simulink model "MYmotoSys1b_centrifugal"  (R2021a)
settings: Solver=ode45  StartTime=0.0  StopTime=20  RelTol=1e-3  EnableMultiTasking=on
PreLoadFcn:
  | moto_cad_data
  | 
  | theta0 = 1;
  | thetadot0 = 0;
undefined symbols (not defined in the file): magnitude, smiData_bike_body, smiData_front_wheel, smiData_reaction_wheel, smiData_rear_wheel, smiData_steer_column, X, Y, Z
libraries: sm_lib x18, nesl_utility x7
settings Model: EnablePacing=on  Creator=smiller  LastModifiedBy=danie
settings SolverCC: AlgebraicLoopSolver=TrustRegion
settings DataIOCC: LimitDataPoints=on  SaveFormat=Array  ReturnWorkspaceOutputs=off
settings OptimizationCC: ExpressionDepthLimit=2147483647  LifeSpan=inf
settings DebuggingCC: UnderspecifiedInitializationDetection=Classic  MergeDetectMultiDrivingBlocksExec=none  ParameterPrecisionLossMsg=none  StateNameClashWarn=warning  SFUnexpectedBacktrackingDiag=warning  SFNoUnconditionalDefaultTransitionDiag=warning  SFExecutionAtInitializationDiag=none  SFMachineParentedDataDiag=warning  ArithmeticOperatorsInVariantConditions=warning
settings HardwareCC: ProdBitPerPointer=32  ProdBitPerSizeT=32  ProdBitPerPtrDiffT=32  ProdLargestAtomicFloat=None  ProdIntDivRoundTo=Undefined  ProdEndianess=Unspecified  ProdWordSize=32  ProdHWDeviceType=32-bit Generic
settings ModelReferenceCC: PropagateSignalLabelsOutOfModel=off
settings SFSimCC: SimUseLocalCustomCode=off  CustomCodeUndefinedFunction=UseInterfaceOnly
settings RTWCC: RTWUseLocalCustomCode=off
settings CodeAppCC: StateflowObjectComments=on
settings GRTTargetCC: TargetLangStandard=C89/C90 (ANSI)
settings ConfigComp: CovMetricSettings=dw  CovSaveCumulativeToWorkspaceVar=on  CovSaveSingleToWorkspaceVar=on  CovExternalEMLEnable=off  CovSFcnEnable=off
settings SimscapeCC: SimscapeNormalizeSystem=off
settings ConfigurationSet: Description=SimMechanics 2G
settings ExplorerConfigSet: InternalSimMechanicsExplorerSettings="<ExplorerConfiguration><canonicalview>default</canonicalview><AnimationSetting><BasePlaybackSpeed>1.0</BasePlaybackSpeed><PlaybackSpeedFactor>1.0</PlaybackSpeedFactor></AnimationSetting><TilePanel><TileInfo><Tiles Columns=\"1\" Count=\"1\" Rows=\"1\"><Column Weight=\"1\"/><Row Weight=\"1\"/><Tile Height=\"1\" Width=\"1\" X=\"0\" Y=\"0\"/></Tiles></TileInfo><SceneInfo><SceneViewer><BGColor><R>0.60000002384185791</R><G>0.60000002384185791</G><B>0.60000002384185791</B></BGColor><Camera><DoPerspective>off</DoPerspective><Position><X>0.918124572942673689</X><Y>-0.460889112225935038</Y><Z>0.271893212526261863</Z></Position><Center><X>0.0428283947711830537</X><Y>-0.012621623404857174</Y><Z>0.090474197689223379</Z></Center><Up><X>-0.135786056615979422</X><Y>0.132236903462622957</Y><Z>0.981873488893196922</Z></Up><ViewLimDist>1</ViewLimDist><YLim>0.105450724735856052</YLim><XLim>0.181023744129886199</XLim></Camera></SceneViewer></SceneInfo></TilePanel><MechEditorPanel><Cameras/><GfxPanelCameraMap/><VideoCreator><PlaybackSpeedRatio>1.0</PlaybackSpeedRatio><FrameRate>30</FrameRate><VideoFormat>Motion JPEG AVI</VideoFormat><FrameSize>auto</FrameSize></VideoCreator></MechEditorPanel></ExplorerConfiguration>"

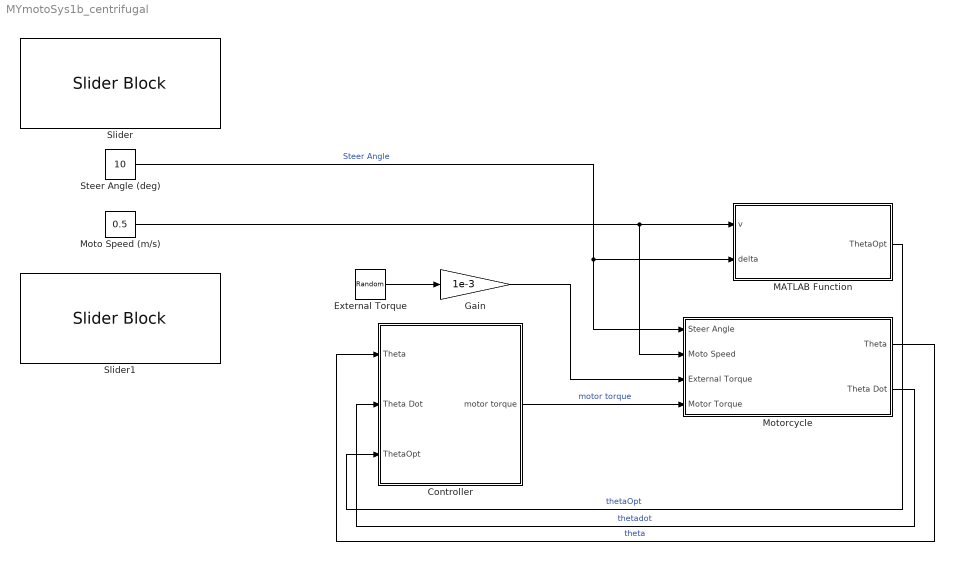
== system MYmotoSys1b_centrifugal ==
  Controller : Subsystem
  External Torque : RandomNumber  SampleTime=0.1
  Gain : Gain  Gain=1e-3
  MATLAB Function : MATLAB Function  TreatAsAtomicUnit=on
  Moto Speed (m/s) : Constant  Value=0.5  SampleTime=-1
  Motorcycle : Subsystem
  Slider : SliderBlock  ScaleMin=-30  ScaleMax=30
  Slider1 : SliderBlock  ScaleMin=-2  ScaleMax=2
  Steer Angle (deg) : Constant  Value=10  SampleTime=-1
  wires:
  Motorcycle/1(Theta) -> Controller/1(Theta)  "theta"
  Motorcycle/2(Theta Dot) -> Controller/2(Theta Dot)  "thetadot"
  External Torque/1 -> Gain/1
  Gain/1 -> Motorcycle/3(External Torque)
  Moto Speed (m/s)/1 -> MATLAB Function/1(v), Motorcycle/2(Moto Speed)
  Steer Angle (deg)/1 -> MATLAB Function/2(delta), Motorcycle/1(Steer Angle)  "Steer Angle"
  Controller/1(motor torque) -> Motorcycle/4(Motor Torque)  "motor torque"
  MATLAB Function/1(ThetaOpt) -> Controller/3(ThetaOpt)  "thetaOpt"

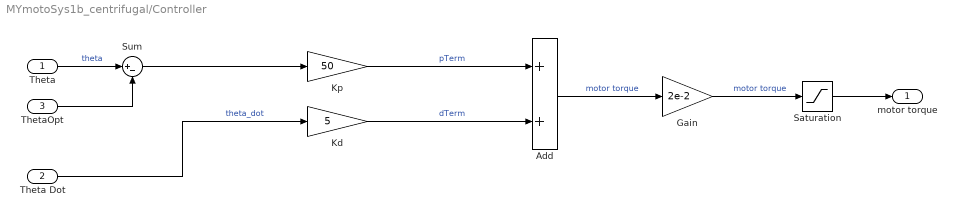
== system MYmotoSys1b_centrifugal/Controller ==
  Theta : Inport
  Theta Dot : Inport  Port=2
  ThetaOpt : Inport  Port=3
  Add : Sum  Inputs=2
  "Gain " : Gain  Gain=2e-2
  Kd : Gain  Gain=5
  Kp : Gain  Gain=50
  Saturation : Saturate  UpperLimit=0.7  LowerLimit=-0.7
  Sum : Sum  Inputs=|+-
  motor torque : Outport  VectorParamsAs1DForOutWhenUnconnected=off
  wires:
  Kd/1 -> Add/2  "dTerm"
  "Gain "/1 -> Saturation/1  "motor torque"
  Kp/1 -> Add/1  "pTerm"
  Theta/1 -> Sum/1  "theta"
  Add/1 -> "Gain "/1  "motor torque"
  Theta Dot/1 -> Kd/1  "theta_dot"
  ThetaOpt/1 -> Sum/2
  Sum/1 -> Kp/1
  Saturation/1 -> motor torque/1

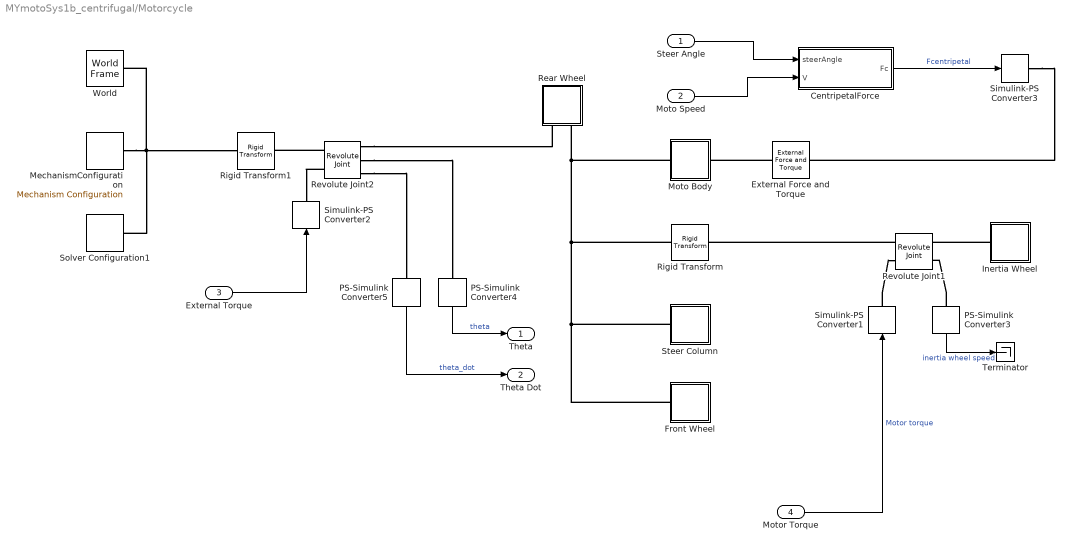
== system MYmotoSys1b_centrifugal/Motorcycle ==
  Steer Angle : Inport
  Moto Speed : Inport  Port=2
  External Torque : Inport  Port=3
  Motor Torque : Inport  Port=4
  CentripetalForce : Subsystem
  External Force and Torque : sm_lib/Forces and Torques/External Force and Torque  ForceResolutionFrame=AttachedFrame  EnableForceX=off  EnableForceY=on  EnableForceZ=off  EnableForce=off  TorqueResolutionFrame=AttachedFrame  EnableTorqueX=off  EnableTorqueY=off  EnableTorqueZ=off  EnableTorque=off
  Front Wheel : Subsystem
  Inertia Wheel : Subsystem
  MechanismConfiguration : sm_lib/Utilities/Mechanism Configuration  UniformGravity=Constant  GravityVector=[0 0 -9.80665]  GravityVectorUnits=m/s^2  GravityUnits=m/s^2  LinearizationDelta=0.001  JointModeTransitionNonlinearIterations=2
  Moto Body : Subsystem
  PS-Simulink Converter3 : nesl_utility/PS-Simulink Converter  PhysicalDomain=network_engine_domain  SubClassName=ps_output  LeftPortType=input  RightPortType=output  PseudoPeriodic=off  Frequencies=[]  Unit=rev/s  AffineConversion=off
      settings: SourceProductBaseCode=PW,SS
  PS-Simulink Converter4 : nesl_utility/PS-Simulink Converter  PhysicalDomain=network_engine_domain  SubClassName=ps_output  LeftPortType=input  RightPortType=output  PseudoPeriodic=off  Frequencies=[]  Unit=deg  AffineConversion=off
      settings: SourceProductBaseCode=PW,SS
  PS-Simulink Converter5 : nesl_utility/PS-Simulink Converter  PhysicalDomain=network_engine_domain  SubClassName=ps_output  LeftPortType=input  RightPortType=output  PseudoPeriodic=off  Frequencies=[]  Unit=deg/s  AffineConversion=off
      settings: SourceProductBaseCode=PW,SS
  Rear Wheel : Subsystem
  Revolute Joint1 : sm_lib/Joints/Revolute Joint  JointMode=Normal  SenseConstraintForce=off  SenseConstraintForceX=off  SenseConstraintForceY=off  SenseConstraintForceZ=off  SenseConstraintTorque=off  SenseConstraintTorqueX=off  SenseConstraintTorqueY=off  SenseConstraintTorqueZ=off  SenseTotalForce=off  SenseTotalForceX=off  SenseTotalForceY=off  SenseTotalForceZ=off  SenseTotalTorque=off  SenseTotalTorqueX=off  SenseTotalTorqueY=off  SenseTotalTorqueZ=off  CompositeWrenchDir=FollowerOnBase  CompositeWrenchFrame=BaseFrame  EquilibriumPosition=0  EquilibriumPositionUnits=deg  SpringStiffness=0  SpringStiffnessUnits=N*m/deg  DampingCoefficient=0  DampingCoefficientUnits=N*m/(deg/s)  TorqueActuationMode=InputTorque  MotionActuationMode=ComputedMotion  SensePosition=off  SenseVelocity=on  SenseAcceleration=off  SenseTorqueForce=off  SenseLowerLimitTorqueForce=off  SenseUpperLimitTorqueForce=off  LowerLimitSpecify=off  LowerLimitBound=-90  LowerLimitBoundUnits=deg  LowerLimitStiffness=1e4  LowerLimitStiffnessUnits=N*m/deg  LowerLimitDamping=10  LowerLimitDampingUnits=N*m/(deg/s)  LowerLimitTransitionRegionWidth=0.1  LowerLimitTransitionRegionWidthUnits=deg  UpperLimitSpecify=off  UpperLimitBound=90  UpperLimitBoundUnits=deg  UpperLimitStiffness=1e4  UpperLimitStiffnessUnits=N*m/deg  UpperLimitDamping=10  UpperLimitDampingUnits=N*m/(deg/s)  UpperLimitTransitionRegionWidth=0.1  UpperLimitTransitionRegionWidthUnits=deg  PositionTargetSpecify=off  PositionTargetPriority=High  PositionTargetValue=0  PositionTargetValueUnits=deg  VelocityTargetSpecify=on  VelocityTargetPriority=High  VelocityTargetValue=0  VelocityTargetValueUnits=deg/s
  Revolute Joint2 : sm_lib/Joints/Revolute Joint  JointMode=Normal  SenseConstraintForce=off  SenseConstraintForceX=off  SenseConstraintForceY=off  SenseConstraintForceZ=off  SenseConstraintTorque=off  SenseConstraintTorqueX=off  SenseConstraintTorqueY=off  SenseConstraintTorqueZ=off  SenseTotalForce=off  SenseTotalForceX=off  SenseTotalForceY=off  SenseTotalForceZ=off  SenseTotalTorque=off  SenseTotalTorqueX=off  SenseTotalTorqueY=off  SenseTotalTorqueZ=off  CompositeWrenchDir=FollowerOnBase  CompositeWrenchFrame=BaseFrame  EquilibriumPosition=0  EquilibriumPositionUnits=deg  SpringStiffness=0  SpringStiffnessUnits=N*m/deg  DampingCoefficient=0  DampingCoefficientUnits=N*m/(deg/s)  TorqueActuationMode=InputTorque  MotionActuationMode=ComputedMotion  SensePosition=on  SenseVelocity=on  SenseAcceleration=off  SenseTorqueForce=off  SenseLowerLimitTorqueForce=off  SenseUpperLimitTorqueForce=off  LowerLimitSpecify=off  LowerLimitBound=-90  LowerLimitBoundUnits=deg  LowerLimitStiffness=1e4  LowerLimitStiffnessUnits=N*m/deg  LowerLimitDamping=10  LowerLimitDampingUnits=N*m/(deg/s)  LowerLimitTransitionRegionWidth=0.1  LowerLimitTransitionRegionWidthUnits=deg  UpperLimitSpecify=off  UpperLimitBound=90  UpperLimitBoundUnits=deg  UpperLimitStiffness=1e4  UpperLimitStiffnessUnits=N*m/deg  UpperLimitDamping=10  UpperLimitDampingUnits=N*m/(deg/s)  UpperLimitTransitionRegionWidth=0.1  UpperLimitTransitionRegionWidthUnits=deg  PositionTargetSpecify=on  PositionTargetPriority=High  PositionTargetValue=theta0  PositionTargetValueUnits=deg  VelocityTargetSpecify=on  VelocityTargetPriority=High  VelocityTargetValue=thetadot0  VelocityTargetValueUnits=deg/s
  Rigid Transform : sm_lib/Frames and Transforms/Rigid Transform  TranslationMethod=Cartesian  TranslationStandardOffset=0  TranslationLengthUnit=mm  TranslationStandardAxis=+Z  TranslationCartesianOffset=[33 -11 126]  TranslationROffset=0  TranslationROffsetUnits=m  TranslationZOffset=0  TranslationZOffsetUnits=m  TranslationThetaOffset=0  TranslationThetaOffsetUnits=deg  RotationMethod=StandardAxis  RotationAngleUnits=deg  RotationStandardAxis=-Y  RotationAngle=90  RotationArbitraryAxis=[0 0 1]  FollAlignAxisA=+X  BaseAlignAxisA=+Y  FollAlignAxisB=+Y  BaseAlignAxisB=+Z  RotationSequenceAxes=FollowerAxes  RotationSequence=XYX  RotationSequenceAngles=[0 0 0]  RotationSequenceAnglesUnits=deg  RotationMatrix=[1 0 0; 0 1 0; 0 0 1]
  Rigid Transform1 : sm_lib/Frames and Transforms/Rigid Transform  TranslationMethod=Cartesian  TranslationStandardOffset=0  TranslationLengthUnit=mm  TranslationStandardAxis=+Z  TranslationCartesianOffset=[150 -11 0]  TranslationROffset=0  TranslationROffsetUnits=m  TranslationZOffset=0  TranslationZOffsetUnits=m  TranslationThetaOffset=0  TranslationThetaOffsetUnits=deg  RotationMethod=StandardAxis  RotationAngleUnits=deg  RotationStandardAxis=-Y  RotationAngle=90  RotationArbitraryAxis=[0 0 1]  FollAlignAxisA=+X  BaseAlignAxisA=+Y  FollAlignAxisB=+Y  BaseAlignAxisB=+Z  RotationSequenceAxes=FollowerAxes  RotationSequence=XYX  RotationSequenceAngles=[0 0 0]  RotationSequenceAnglesUnits=deg  RotationMatrix=[1 0 0; 0 1 0; 0 0 1]
  Simulink-PS Converter1 : nesl_utility/Simulink-PS Converter  PhysicalDomain=network_engine_domain  SubClassName=ps_input  LeftPortType=input  RightPortType=output  PseudoPeriodic=off  Frequencies=[]  NoiseDistribution=none  NoiseParameters=[]  Unit=N*m  AffineConversion=off  FilteringAndDerivatives=provide  SimscapeFilterOrder=1  InputFilterTimeConstant=0.001  UdotUserProvided=0
      settings: SourceProductBaseCode=PW,SS
  Simulink-PS Converter2 : nesl_utility/Simulink-PS Converter  PhysicalDomain=network_engine_domain  SubClassName=ps_input  LeftPortType=input  RightPortType=output  PseudoPeriodic=off  Frequencies=[]  NoiseDistribution=none  NoiseParameters=[]  Unit=N*m  AffineConversion=off  FilteringAndDerivatives=provide  SimscapeFilterOrder=1  InputFilterTimeConstant=0.001  UdotUserProvided=0
      settings: SourceProductBaseCode=PW,SS
  Simulink-PS Converter3 : nesl_utility/Simulink-PS Converter  PhysicalDomain=network_engine_domain  SubClassName=ps_input  LeftPortType=input  RightPortType=output  PseudoPeriodic=off  Frequencies=[]  NoiseDistribution=none  NoiseParameters=[]  Unit=N  AffineConversion=off  FilteringAndDerivatives=provide  SimscapeFilterOrder=1  InputFilterTimeConstant=0.001  UdotUserProvided=0
      settings: SourceProductBaseCode=PW,SS
  Solver Configuration1 : nesl_utility/Solver Configuration  PhysicalDomain=network_engine_domain  SubClassName=solver  LeftPortType=input  RightPortType=generic  Tones=[]  Harmonics=[]  SimulateNoise=off  Profile=off  UseLocalSampling=off  EnableSwitchedLinearOptims=on  FrequencyDomain=off  UseCCode=off  RelTol=0.001  AbsTol=1e-06  MinStep=1e-09  ToWorkspace=off  RevertToSquareIcSolve=off  NumHomotopyIterations=100  PhasorMode=off  PhasorModeNumHarmonics=1  DoDC=off  ResidualTolerance=1e-09  UseLocalSolver=off  LocalSolverChoice=NE_BACKWARD_EULER_ADVANCER  LocalSolverSampleTime=0.001  DoFixedCost=off  MaxNonlinIter=3  MaxModeIter=2  ComputeImpulses=off  ImpulseIterations=2  LinearAlgebra=Sparse  EquationFormulation=NE_TIME_EF  DelaysMemoryBudget=1024  AutomaticFiltering=on  FilteringTimeConstant=0.001  PartitionStorageMethod=AS_NEEDED  PartitionMemoryBudget=1024  PartitionMethod=FAST
      settings: SourceProductBaseCode=PW,SS
  Steer Column : Subsystem
  Terminator : Terminator
  World : sm_lib/Frames and Transforms/World Frame
  Theta : Outport  VectorParamsAs1DForOutWhenUnconnected=off
  Theta Dot : Outport  Port=2  VectorParamsAs1DForOutWhenUnconnected=off
  wires:
  PS-Simulink Converter4/1 -> Theta/1  "theta"
  PS-Simulink Converter5/1 -> Theta Dot/1  "theta_dot"
  External Torque/1 -> Simulink-PS Converter2/1
  Motor Torque/1 -> Simulink-PS Converter1/1  "Motor torque"
  PS-Simulink Converter3/1 -> Terminator/1  "inertia wheel speed"
  Steer Angle/1 -> CentripetalForce/1(steerAngle)
  Moto Speed/1 -> CentripetalForce/2(V)
  CentripetalForce/1(Fc) -> Simulink-PS Converter3/1  "Fcentripetal"
  connections:
  Front Wheel/LConn1 -- Steer Column/LConn1 -- Rear Wheel/LConn2 -- Moto Body/LConn1 -- Rigid Transform/LConn1
  MechanismConfiguration/RConn1 -- Solver Configuration1/RConn1 -- Rigid Transform1/LConn1 -- World/RConn1
  Revolute Joint1/LConn1 -- Rigid Transform/RConn1
  Revolute Joint2/RConn2 -- PS-Simulink Converter4/LConn1
  Revolute Joint2/LConn1 -- Rigid Transform1/RConn1
  Revolute Joint2/LConn2 -- Simulink-PS Converter2/RConn1
  PS-Simulink Converter3/LConn1 -- Revolute Joint1/RConn2
  Inertia Wheel/LConn1 -- Revolute Joint1/RConn1
  Revolute Joint2/RConn1 -- Rear Wheel/LConn1
  Simulink-PS Converter1/RConn1 -- Revolute Joint1/LConn2
  Revolute Joint2/RConn3 -- PS-Simulink Converter5/LConn1
  Simulink-PS Converter3/RConn1 -- External Force and Torque/LConn1
  External Force and Torque/RConn1 -- Moto Body/RConn1

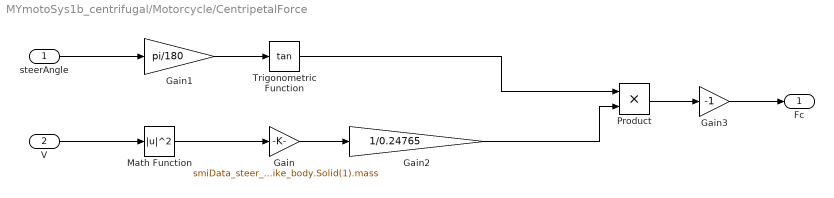
== system MYmotoSys1b_centrifugal/Motorcycle/CentripetalForce ==
  steerAngle : Inport
  V : Inport  Port=2
  Gain : Gain  Gain=smiData_steer_column.Solid(1).mass+smiData_rear_wheel.Solid(1).mass+smiData_front_wheel.Solid(1).mass+smiData_reaction_wheel.Solid(1).mass+smiData_bike_body.Solid(1).mass
  Gain1 : Gain  Gain=pi/180
  Gain2 : Gain  Gain=1/0.24765
  Gain3 : Gain  Gain=-1
  Math Function : Math  Operator=magnitude^2  SignedPower=on  SaturateOnIntegerOverflow=on
  Product : Product
  Trigonometric Function : Trigonometry  Operator=tan
  Fc : Outport  VectorParamsAs1DForOutWhenUnconnected=off
  wires:
  V/1 -> Math Function/1
  steerAngle/1 -> Gain1/1
  Math Function/1 -> Gain/1
  Gain/1 -> Gain2/1
  Gain1/1 -> Trigonometric Function/1
  Gain2/1 -> Product/2
  Product/1 -> Gain3/1
  Trigonometric Function/1 -> Product/1
  Gain3/1 -> Fc/1

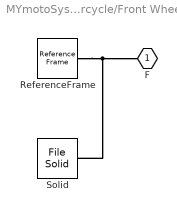
== system MYmotoSys1b_centrifugal/Motorcycle/Front Wheel ==
  ReferenceFrame : sm_lib/Frames and Transforms/Reference Frame
  Solid : sm_lib/Body Elements/File Solid  ExtGeomFileName=MotorcycleLowpolyRhino4_front_wheel_Default_sldprt.STEP  UnitType=FromFile  ExtGeomFileUnits=m  StepReaderType=HEX  ExportConvexHullGeometry=off  InertiaType=Custom  Mass=smiData_front_wheel.Solid(1).mass  MassUnits=kg  CenterOfMass=smiData_front_wheel.Solid(1).CoM  CenterOfMassUnits=mm  MomentsOfInertia=smiData_front_wheel.Solid(1).MoI  MomentsOfInertiaUnits=kg*mm^2  ProductsOfInertia=smiData_front_wheel.Solid(1).PoI  ProductsOfInertiaUnits=kg*mm^2  BasedOnType=Density  Density=1000  DensityUnits=kg/m^3  DoExposeReferenceFrame=on  SerializedFrames=<Frames/>  GraphicType=FromGeometry  MarkerShape=Sphere  MarkerSize=10  GraphicVisPropType=SimpleVisualProperties  GraphicDiffuseColor=[0.4 0.4 0.4]  GraphicSpecularColor=[0.5 0.5 0.5 1.0]  GraphicAmbientColor=[0.15 0.15 0.15 1.0]  GraphicEmissiveColor=[0.0 0.0 0.0 1.0]  GraphicShininess=75  GraphicOpacity=smiData_front_wheel.Solid(1).opacity
  F : PMIOPort  Side=Left
  connections:
  Solid/RConn1 -- ReferenceFrame/RConn1 -- F/RConn1

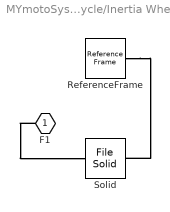
== system MYmotoSys1b_centrifugal/Motorcycle/Inertia Wheel ==
  ReferenceFrame : sm_lib/Frames and Transforms/Reference Frame
  Solid : sm_lib/Body Elements/File Solid  ExtGeomFileName=MotorcycleLowpolyRhino4_reaction_wheel_Default_sldprt.STEP  UnitType=FromFile  ExtGeomFileUnits=m  StepReaderType=OCC  ExportConvexHullGeometry=off  InertiaType=Custom  Mass=smiData_reaction_wheel.Solid(1).mass  MassUnits=kg  CenterOfMass=smiData_reaction_wheel.Solid(1).CoM  CenterOfMassUnits=mm  MomentsOfInertia=smiData_reaction_wheel.Solid(1).MoI  MomentsOfInertiaUnits=kg*mm^2  ProductsOfInertia=smiData_reaction_wheel.Solid(1).PoI  ProductsOfInertiaUnits=kg*mm^2  BasedOnType=Density  Density=1000  DensityUnits=kg/m^3  DoExposeReferenceFrame=on  SerializedFrames=<Frames><Frame><Id>Frame1</Id><Value><Name>F1</Name><Origin><Source>CenterOfMassFrame</Source><FeatureName></FeatureName></Origin><PrimaryAxis><DefinedDirection>+Z</DefinedDirection><Source>GeometricFeature</Source><SourceDirection>+Z</SourceDirection><FeatureName>planar surface 3</FeatureName></PrimaryAxis><SecondaryAxis><DefinedDirection>+Y</DefinedDirection><Source>GeometricFeature</Source><SourceDirection>+X</SourceDirection><FeatureName>planar surface 4</FeatureName></SecondaryAxis></Value></Frame></Frames>  GraphicType=FromGeometry  MarkerShape=Sphere  MarkerSize=10  GraphicVisPropType=SimpleVisualProperties  GraphicDiffuseColor=[1.0 0.0 0.2]  GraphicSpecularColor=[0.5 0.5 0.5 1.0]  GraphicAmbientColor=[0.15 0.15 0.15 1.0]  GraphicEmissiveColor=[0.0 0.0 0.0 1.0]  GraphicShininess=75  GraphicOpacity=smiData_reaction_wheel.Solid(1).opacity
  F1 : PMIOPort  Side=Left
  connections:
  ReferenceFrame/RConn1 -- Solid/RConn1
  F1/RConn1 -- Solid/LConn1

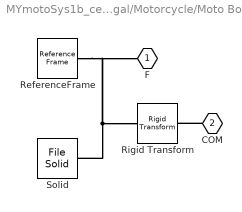
== system MYmotoSys1b_centrifugal/Motorcycle/Moto Body ==
  ReferenceFrame : sm_lib/Frames and Transforms/Reference Frame
  Rigid Transform : sm_lib/Frames and Transforms/Rigid Transform  TranslationMethod=Cartesian  TranslationStandardOffset=0  TranslationLengthUnit=mm  TranslationStandardAxis=+Z  TranslationCartesianOffset=(smiData_bike_body.Solid.mass*smiData_bike_body.Solid.CoM+smiData_rear_wheel.Solid.mass*smiData_rear_wheel.Solid.CoM+smiData_front_wheel.Solid.mass*smiData_front_wheel.Solid.CoM+smiData_reaction_wheel.Solid.mass*smiData_reaction_wheel.Solid.CoM+smiData_steer_column.Solid.mass*smiData_steer_column.Solid.CoM)/(smiData_bike_body.Solid.mass+smiData_rear_wheel.Solid.mass+smiData_front_wheel.Solid.mass+smiData_reaction_wheel.Solid.mass+smiData_steer_column.Solid.mass)  TranslationROffset=0  TranslationROffsetUnits=m  TranslationZOffset=0  TranslationZOffsetUnits=m  TranslationThetaOffset=0  TranslationThetaOffsetUnits=deg  RotationMethod=None  RotationAngleUnits=deg  RotationStandardAxis=+Z  RotationAngle=0.0  RotationArbitraryAxis=[0 0 1]  FollAlignAxisA=+X  BaseAlignAxisA=+Y  FollAlignAxisB=+Y  BaseAlignAxisB=+Z  RotationSequenceAxes=FollowerAxes  RotationSequence=XYX  RotationSequenceAngles=[0 0 0]  RotationSequenceAnglesUnits=deg  RotationMatrix=[1 0 0; 0 1 0; 0 0 1]
  Solid : sm_lib/Body Elements/File Solid  ExtGeomFileName=MotorcycleLowpolyRhino4_bike_body_Default_sldprt.STEP  UnitType=FromFile  ExtGeomFileUnits=m  StepReaderType=HEX  ExportConvexHullGeometry=off  InertiaType=Custom  Mass=smiData_bike_body.Solid(1).mass  MassUnits=kg  CenterOfMass=smiData_bike_body.Solid(1).CoM  CenterOfMassUnits=mm  MomentsOfInertia=smiData_bike_body.Solid(1).MoI  MomentsOfInertiaUnits=kg*mm^2  ProductsOfInertia=smiData_bike_body.Solid(1).PoI  ProductsOfInertiaUnits=kg*mm^2  BasedOnType=Density  Density=1000  DensityUnits=kg/m^3  DoExposeReferenceFrame=on  SerializedFrames=<Frames/>  GraphicType=FromGeometry  MarkerShape=Sphere  MarkerSize=10  GraphicVisPropType=SimpleVisualProperties  GraphicDiffuseColor=[0.0 0.6 0.6]  GraphicSpecularColor=[0.5 0.5 0.5 1.0]  GraphicAmbientColor=[0.15 0.15 0.15 1.0]  GraphicEmissiveColor=[0.0 0.0 0.0 1.0]  GraphicShininess=75  GraphicOpacity=smiData_bike_body.Solid(1).opacity
  F : PMIOPort  Side=Left
  COM : PMIOPort  Port=2  Side=Right
  connections:
  ReferenceFrame/RConn1 -- F/RConn1 -- Solid/RConn1 -- Rigid Transform/LConn1
  COM/RConn1 -- Rigid Transform/RConn1

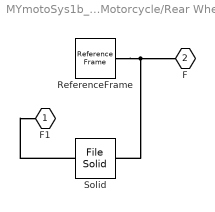
== system MYmotoSys1b_centrifugal/Motorcycle/Rear Wheel ==
  ReferenceFrame : sm_lib/Frames and Transforms/Reference Frame
  Solid : sm_lib/Body Elements/File Solid  ExtGeomFileName=MotorcycleLowpolyRhino4_rear_wheel_Default_sldprt.STEP  UnitType=FromFile  ExtGeomFileUnits=m  StepReaderType=OCC  ExportConvexHullGeometry=off  InertiaType=Custom  Mass=smiData_rear_wheel.Solid(1).mass  MassUnits=kg  CenterOfMass=smiData_rear_wheel.Solid(1).CoM  CenterOfMassUnits=mm  MomentsOfInertia=smiData_rear_wheel.Solid(1).MoI  MomentsOfInertiaUnits=kg*mm^2  ProductsOfInertia=smiData_rear_wheel.Solid(1).PoI  ProductsOfInertiaUnits=kg*mm^2  BasedOnType=Density  Density=1000  DensityUnits=kg/m^3  DoExposeReferenceFrame=on  SerializedFrames=<Frames><Frame><Id>Frame1</Id><Value><Name>F1</Name><Origin><Source>GeometricFeature</Source><FeatureName>segment 92</FeatureName></Origin><PrimaryAxis><DefinedDirection>-Y</DefinedDirection><Source>GeometricFeature</Source><SourceDirection>+Z</SourceDirection><FeatureName>segment 92</FeatureName></PrimaryAxis><SecondaryAxis><DefinedDirection>-Z</DefinedDirection><Source>GeometricFeature</Source><SourceDirection>+X</SourceDirection><FeatureName>planar surface 20</FeatureName></SecondaryAxis></Value></Frame></Frames>  GraphicType=FromGeometry  MarkerShape=Sphere  MarkerSize=10  GraphicVisPropType=SimpleVisualProperties  GraphicDiffuseColor=[0.4 0.4 0.4]  GraphicSpecularColor=[0.5 0.5 0.5 1.0]  GraphicAmbientColor=[0.15 0.15 0.15 1.0]  GraphicEmissiveColor=[0.0 0.0 0.0 1.0]  GraphicShininess=75  GraphicOpacity=smiData_rear_wheel.Solid(1).opacity
  F1 : PMIOPort  Side=Left
  F : PMIOPort  Port=2  Side=Left
  connections:
  Solid/RConn1 -- ReferenceFrame/RConn1 -- F/RConn1
  Solid/LConn1 -- F1/RConn1

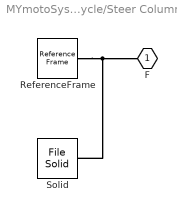
== system MYmotoSys1b_centrifugal/Motorcycle/Steer Column ==
  ReferenceFrame : sm_lib/Frames and Transforms/Reference Frame
  Solid : sm_lib/Body Elements/File Solid  ExtGeomFileName=MotorcycleLowpolyRhino4_steer_column_Default_sldprt.STL  UnitType=Custom  ExtGeomFileUnits=mm  StepReaderType=HEX  ExportConvexHullGeometry=off  InertiaType=Custom  Mass=smiData_steer_column.Solid(1).mass  MassUnits=kg  CenterOfMass=smiData_steer_column.Solid(1).CoM  CenterOfMassUnits=mm  MomentsOfInertia=smiData_steer_column.Solid(1).MoI  MomentsOfInertiaUnits=kg*mm^2  ProductsOfInertia=smiData_steer_column.Solid(1).PoI  ProductsOfInertiaUnits=kg*mm^2  BasedOnType=Density  Density=1000  DensityUnits=kg/m^3  DoExposeReferenceFrame=on  SerializedFrames=<Frames/>  GraphicType=FromGeometry  MarkerShape=Sphere  MarkerSize=10  GraphicVisPropType=SimpleVisualProperties  GraphicDiffuseColor=[0.0 0.2 0.8]  GraphicSpecularColor=[0.5 0.5 0.5 1.0]  GraphicAmbientColor=[0.15 0.15 0.15 1.0]  GraphicEmissiveColor=[0.0 0.0 0.0 1.0]  GraphicShininess=75  GraphicOpacity=smiData_steer_column.Solid(1).opacity
  F : PMIOPort  Side=Left
  connections:
  ReferenceFrame/RConn1 -- Solid/RConn1 -- F/RConn1

== matlab function MYmotoSys1b_centrifugal/MATLAB Function ==
  data: v input; ThetaOpt output; delta input
function ThetaOpt = ThetaOpt_fcn(v,delta)
g=9.81;
L_FR=0.25;
ThetaOpt =atand((v^2*delta)/(g*L_FR));
